simulink subsystem "PvtSubSys_VSM_ELK"  (R2020b)
settings: Solver=VariableStepAuto  StartTime=0.0  StopTime=10.0  RelTol=1e-3
values from neighbouring files (symbols this model uses):
  P_VSM_ELK_Curvature_R_Table : value not decoded    [ELK.sldd]
  P_VSM_ELK_Curvature_R_Table_Calibration : value not decoded    [ELK.sldd]
  P_VSM_ELK_Lane_Width_Table : value not decoded    [ELK.sldd]
  P_VSM_ELK_Lane_Width_Table_Calibration : value not decoded    [ELK.sldd]
  P_VSM_ELK_Lateral_Speed_Table : value not decoded    [ELK.sldd]
  P_VSM_ELK_Lateral_Speed_Table_Calibration : value not decoded    [ELK.sldd]
  P_VSM_ELK_OnComing_Lateral = 2.8    [ELK.sldd]
  P_VSM_ELK_OnComing_TTC = 3.0    [ELK.sldd]
  P_VSM_ELK_OverTaking_Lateral = 2.0    [ELK.sldd]
  P_VSM_ELK_OverTaking_TTC = 5.0    [ELK.sldd]
  P_VSM_ELK_Sensitive_Table : value not decoded    [ELK.sldd]
  P_VSM_ELK_Sensitive_Table_Calibration : value not decoded    [ELK.sldd]
  P_VSM_ELK_State_Absesp_enable = 1.0    [ELK.sldd]
  P_VSM_ELK_State_Accpedalrate_enable = 1.0    [ELK.sldd]
  P_VSM_ELK_State_Breakpressure_enable = 1.0    [ELK.sldd]
  P_VSM_ELK_State_DriverInputTrqValue_enable = 1.0    [ELK.sldd]
  P_VSM_ELK_State_Eps_enable = 1.0    [ELK.sldd]
  P_VSM_ELK_State_ESSSts_enable = 1.0    [ELK.sldd]
  P_VSM_ELK_State_Failsafe_enable = 1.0    [ELK.sldd]
  P_VSM_ELK_State_GEAR_enable = 1.0    [ELK.sldd]
  P_VSM_ELK_State_Handson_enable = 1.0    [ELK.sldd]
  P_VSM_ELK_State_Headingangle_enable = 1.0    [ELK.sldd]
  P_VSM_ELK_State_Lane_enable = 1.0    [ELK.sldd]
  P_VSM_ELK_State_LaneChange_enable = 1.0    [ELK.sldd]
  P_VSM_ELK_State_Lanecurve_enable = 1.0    [ELK.sldd]
  P_VSM_ELK_State_LateralAcce_enable = 1.0    [ELK.sldd]
  P_VSM_ELK_State_LongitudeAcc_enable = 1.0    [ELK.sldd]
  P_VSM_ELK_State_Overide_enable = 1.0    [ELK.sldd]
  P_VSM_ELK_State_Param_AngleOffset = 0.05    [ELK.sldd]
  P_VSM_ELK_State_Param_LaneTime : value not decoded    [ELK.sldd]
  P_VSM_ELK_State_Param_Oncoming = 0.55    [ELK.sldd]
  P_VSM_ELK_State_Param_OnTime : value not decoded    [ELK.sldd]
  P_VSM_ELK_State_Param_OutOffset = 0.15    [ELK.sldd]
  P_VSM_ELK_State_Param_Over = 0.55    [ELK.sldd]
  P_VSM_ELK_State_Param_OvTime : value not decoded    [ELK.sldd]
  P_VSM_ELK_State_Param_Speed : value not decoded    [ELK.sldd]
  P_VSM_ELK_State_SteerWheelAngle_enable = 1.0    [ELK.sldd]
  P_VSM_ELK_State_SteerWheelSpd_enable = 1.0    [ELK.sldd]
  P_VSM_ELK_State_TurnLight_enable = 1.0    [ELK.sldd]
  P_VSM_ELK_State_Vehspeed_enable = 1.0    [ELK.sldd]
  P_VSM_ELK_State_Yawsup_enable = 1.0    [ELK.sldd]
undefined symbols (not defined in the file or in its folder): ELKSTATE, P_Global_DxvRearBumper_m, P_Global_IEnvironment_RefPX_Front_Bumper, P_Global_IFV2Fwheel_Dx, P_Global_Vehicle_Length_m, P_Global_VehicleWidthMin_m, P_VSM_LSMC_SampleTime
libraries: simulink x167
(part 4 of 5)

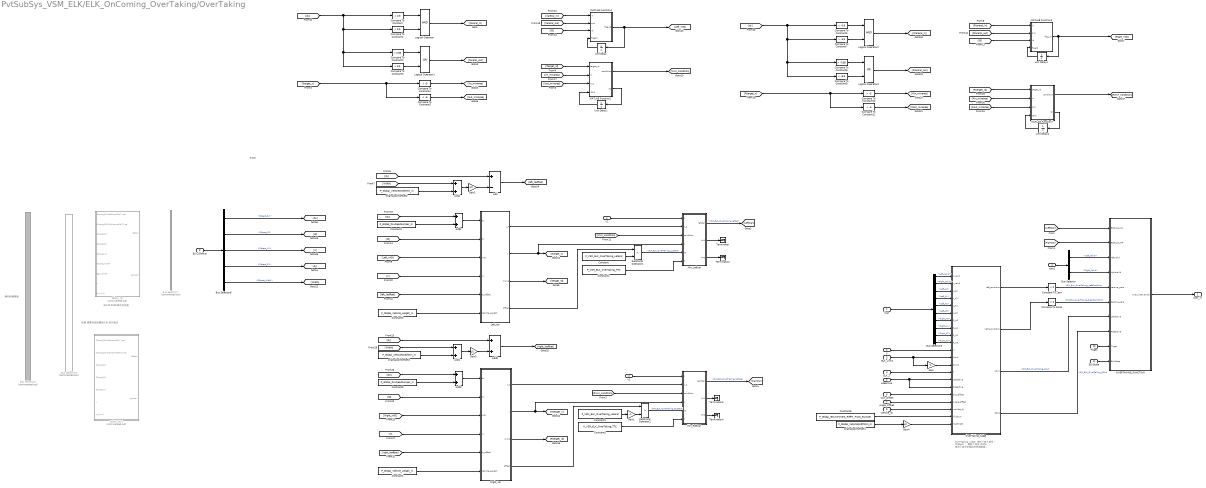
== system PvtSubSys_VSM_ELK/ELK_OnComing_OverTaking/OverTaking ==
  note: RSDS
  note: 横向距离限制
  note: 未对ttc和dtc做冗余处理
  note: 后期 需要对目标属性正负 进行验证
  note: OverTaking_Judge
      | 增加了输入信号：
      | ifv2bum；
      | 删除了信号
      | ifv2fw
      | 修改了自车车辆动态预测距离；
  ican : Inport
  V : Inport  Port=2
  ELK_Limit : Inport  Port=3
  ELK_T : Inport  Port=4
  Ldeactive : Inport  Port=5
  Out_Offset : Inport  Port=6
  Angle_Offset : Inport  Port=7
  ELK_ObjBus : Inport  Port=8
  Vehicle_dy : Inport  Port=9
  Triger : Inport  Port=10
  ELKState : Inport  Port=11
  Add : Sum  Inputs=+-
  Add{1..4,6} (5 alike) : Sum
  Bus Selector : BusSelector  OutputSignals=Left_Valid,Right_Valid
  Bus Selector3 : BusSelector  OutputSignals=Left_Valid,Right_Valid,Left_A0,Left_A1,Left_A2,Left_A3,Right_A0,Right_A1,Right_A2,Right_A3
  Bus Selector5 : BusSelector  Commented=on  OutputSignals=RSDSDx_RL,RSDSID_RL,RSDSV_RL,RSDSDy_RL,RSDSWth_RL,RSDSDx_RR,RSDSID_RR,RSDSV_RR,RSDSDy_RR,RSDSWth_RR
  Bus Selector6 : BusSelector  Commented=on  OutputSignals=ELK_Object_DX,ELK_Object_ID,ELK_Object_VX,ELK_Object_DY,ELK_Object_Width,ELK_Object_DX,ELK_Object_ID,ELK_Object_VX,ELK_Object_DY,ELK_Object_Width
  Bus Selector7 : BusSelector  Commented=on  OutputSignals=ELK_Object_DX,ELK_Object_ID,ELK_Object_VX,ELK_Object_DY,ELK_Object_Width
  Bus Selector8 : BusSelector  OutputSignals=Object_DX,Object_ID,Object_VX,Object_DY,Object_Width
  Compare To Constant : simulink/Logic and Bit Operations/Compare To Constant  relop=>  const=0.9  OutDataTypeStr=boolean
  Compare To Constant1 : simulink/Logic and Bit Operations/Compare To Constant  relop=<  const=5.5  OutDataTypeStr=boolean
  Compare To Constant10 : simulink/Logic and Bit Operations/Compare To Constant  relop=>  const=-5  OutDataTypeStr=boolean
  Compare To Constant11 : simulink/Logic and Bit Operations/Compare To Constant  relop=<  const=-6  OutDataTypeStr=boolean
  Compare To Constant2 : simulink/Logic and Bit Operations/Compare To Constant  relop=<  const=0.85  OutDataTypeStr=boolean
  Compare To Constant3 : simulink/Logic and Bit Operations/Compare To Constant  relop=>  const=6.5  OutDataTypeStr=boolean
  Compare To Constant4 : simulink/Logic and Bit Operations/Compare To Constant  relop=>  const=-5  OutDataTypeStr=boolean
  Compare To Constant5 : simulink/Logic and Bit Operations/Compare To Constant  relop=<  const=-6  OutDataTypeStr=boolean
  Compare To Constant6 : simulink/Logic and Bit Operations/Compare To Constant  relop=<  const=-0.9  OutDataTypeStr=boolean
  Compare To Constant7 : simulink/Logic and Bit Operations/Compare To Constant  relop=>  const=-5.5  OutDataTypeStr=boolean
  Compare To Constant8 : simulink/Logic and Bit Operations/Compare To Constant  relop=>  const=-0.85  OutDataTypeStr=boolean
  Compare To Constant9 : simulink/Logic and Bit Operations/Compare To Constant  relop=<  const=-6.5  OutDataTypeStr=boolean
  Compare To Zero : simulink/Logic and Bit Operations/Compare To Zero  relop=<  OutDataTypeStr=boolean
  Compare To Zero1 : simulink/Logic and Bit Operations/Compare To Zero  relop=>  OutDataTypeStr=boolean
  Constant : Constant  Value=P_VSM_ELK_OverTaking_Lateral
  Constant1 : Constant  Value=P_Global_Vehicle_Length_m
  Constant2 : Constant  Value=P_VSM_ELK_OverTaking_Lateral
  Constant3 : Constant  Value=P_Global_Vehicle_Length_m
  Constant4 : Constant  Value=P_VSM_ELK_OverTaking_TTC
  Constant5 : Constant  Value=P_VSM_ELK_OverTaking_TTC
  Constant6 : Constant  Value=P_Global_IEnvironment_RefPX_Front_Bumper
  Constant7 : Constant  Value=P_Global_DxvRearBumper_m
  Constant8 : Constant  Value=P_Global_DxvRearBumper_m
  Gain : Gain  Gain=-1
  Gain1 : Gain  Gain=-1
  Gain2 : Gain  Gain=1/2
  Gain3 : Gain  Gain=1/2
  Gain4 : Gain  Gain=1/2
  Left_tar : MATLAB Function  TreatAsAtomicUnit=on
  Logical Operator : Logic  AllPortsSameDT=off  OutDataTypeStr=boolean
  Logical Operator1 : Logic  Operator=OR  AllPortsSameDT=off  OutDataTypeStr=boolean
  Logical Operator2 : Logic  AllPortsSameDT=off  OutDataTypeStr=boolean
  Logical Operator3 : Logic  Operator=OR  AllPortsSameDT=off  OutDataTypeStr=boolean
  MATLAB Function1 : MATLAB Function  TreatAsAtomicUnit=on
  MATLAB Function3 : MATLAB Function  TreatAsAtomicUnit=on
  MATLAB Function4 : MATLAB Function  TreatAsAtomicUnit=on
  MATLAB Function7 : MATLAB Function  TreatAsAtomicUnit=on
  Min_Leftcar : MATLAB Function  TreatAsAtomicUnit=on
  Min_Reftcar : MATLAB Function  TreatAsAtomicUnit=on
  OVERTAKING_FUNCTION : Stateflow chart  TreatAsAtomicUnit=on
  OverTaking_Judge : MATLAB Function  TreatAsAtomicUnit=on
  Relational Operator1 : RelationalOperator  Operator=<  OutDataTypeStr=boolean  RndMeth=Simplest
  Relational Operator2 : RelationalOperator  Operator=>  OutDataTypeStr=boolean  RndMeth=Simplest
  Right_tar : MATLAB Function  TreatAsAtomicUnit=on
  Select_tar : MATLAB Function  Commented=on  TreatAsAtomicUnit=on
  Select_tar2 : MATLAB Function  Commented=on  TreatAsAtomicUnit=on
  Terminator{,2..4} (4 alike) : Terminator
  Unit Delay{,1..2,4} (4 alike) : UnitDelay  InitialCondition=uint8(0)  SampleTime=-1  HasFrameUpgradeWarning=on
  V1 : InportShadow  Port=2
  V2 : InportShadow  Port=2
  ican1 : InportShadow
  originalpointoffset1 : Constant  Value=P_Global_VehicleWidthMin_m
  originalpointoffset2 : Constant  Value=P_Global_VehicleWidthMin_m
  originalpointoffset3 : Constant  Value=P_Global_VehicleWidthMin_m
  "over_in " : Outport
  wires:
  Bus Selector/2 -> OVERTAKING_FUNCTION/4(rightvalid)  "<Right_Valid>"
  Bus Selector/1 -> OVERTAKING_FUNCTION/3(leftvalid)  "<Left_Valid>"
  ican1/1 -> Bus Selector/1
  Bus Selector3/10 -> OverTaking_Judge/10(R_A3)  "<Right_A3>"
  Bus Selector3/9 -> OverTaking_Judge/9(R_A2)  "<Right_A2>"
  Bus Selector3/8 -> OverTaking_Judge/8(R_A1)  "<Right_A1>"
  Bus Selector3/7 -> OverTaking_Judge/7(R_A0)  "<Right_A0>"
  Bus Selector3/6 -> OverTaking_Judge/6(L_A3)  "<Left_A3>"
  Bus Selector3/5 -> OverTaking_Judge/5(L_A2)  "<Left_A2>"
  Bus Selector3/4 -> OverTaking_Judge/4(L_A1)  "<Left_A1>"
  Bus Selector3/3 -> OverTaking_Judge/3(L_A0)  "<Left_A0>"
  Bus Selector3/2 -> OverTaking_Judge/2(r_valid)  "<Right_Valid>"
  Bus Selector3/1 -> OverTaking_Judge/1(l_valid)  "<Left_Valid>"
  Gain3/1 -> Add6/2
  [Width] -> Add1/1
  [V] -> Right_tar/4(vx)
  [Dx] -> Add3/1
  [dy] -> Add6/1
  [ID] -> Right_tar/2(id)
  [V] -> Left_tar/4(vx)
  Bus Selector8/3 -> [V]  "<Object_VX>"
  [Dx] -> Add2/1
  Bus Selector8/1 -> [Dx]  "<Object_DX>"
  [ID] -> Left_tar/2(id)
  Bus Selector8/2 -> [ID]  "<Object_ID>"
  [Width] -> Add4/1
  Bus Selector8/5 -> [Width]  "<Object_Width>"
  Bus Selector8/4 -> [dy]  "<Object_DY>"
  Unit Delay2/1 -> MATLAB Function7/4(IDk1)
  MATLAB Function7/2(ID) -> Unit Delay2/1
  Unit Delay1/1 -> MATLAB Function1/4(IDk1)
  MATLAB Function1/2(ID) -> Unit Delay1/1
  Unit Delay/1 -> MATLAB Function4/4(flagk1)
  MATLAB Function4/1(flag_id) -> Unit Delay/1, [Left_inID]
  Unit Delay4/1 -> MATLAB Function3/4(flagk1)
  Gain1/1 -> Relational Operator2/2
  Constant2/1 -> Gain1/1
  Constant/1 -> Relational Operator1/2
  Angle_Offset/1 -> OverTaking_Judge/18(Angle_Offset)
  Out_Offset/1 -> OverTaking_Judge/17(Out_Offset)
  OverTaking_Judge/4(ROut) -> OVERTAKING_FUNCTION/8(Rdeactive)  "VSM_ELK_OverTaking_ROut"
  OverTaking_Judge/3(LOut) -> OVERTAKING_FUNCTION/7(Ldeactive)  "VSM_ELK_OverTaking_LOut"
  OverTaking_Judge/2(right_condition) -> Compare To Zero1/1
  OverTaking_Judge/1(left_condition) -> Compare To Zero/1
  [right_laoffset] -> Right_tar/5(la_offset)
  [left_laoffset] -> Left_tar/5(la_offset)
  Relational Operator2/1 -> Min_Reftcar/5(la)  "VSM_ELK_OverTaking_RLateral"
  Right_tar/4(offset) -> Relational Operator2/1
  Relational Operator1/1 -> Min_Leftcar/5(la)  "VSM_ELK_OverTaking_LLateral"
  Left_tar/4(offset) -> Relational Operator1/1
  Add6/1 -> [right_laoffset]
  Add1/1 -> Gain3/1
  Add/1 -> [left_laoffset]
  Constant8/1 -> Add3/2
  Add3/1 -> Right_tar/1(dx)
  Constant3/1 -> Left_tar/6(Vehicle_Length)
  Add2/1 -> Left_tar/1(dx)
  [ID] -> MATLAB Function3/3(id)
  Compare To Constant6/1 -> Logical Operator2/1
  [Rin_minarea] -> MATLAB Function7/2(in)
  MATLAB Function3/1(flag_id) -> Unit Delay4/1, [Right_inID]
  [Rterget_id] -> MATLAB Function7/1(target_id)
  [Rout_minarea] -> MATLAB Function7/3(out)
  MATLAB Function7/1(condition) -> [Rmin_condition]
  Compare To Constant7/1 -> Logical Operator2/2
  Compare To Constant9/1 -> Logical Operator3/2
  Logical Operator2/1 -> [Rlareral_in]
  Compare To Constant11/1 -> [Rout_minarea]
  Compare To Constant8/1 -> Logical Operator3/1
  [Rterget_x] -> Compare To Constant11/1, Compare To Constant10/1
  [dy] -> Compare To Constant9/1, Compare To Constant8/1, Compare To Constant7/1, Compare To Constant6/1
  Logical Operator3/1 -> [Rlareral_out]
  Compare To Constant10/1 -> [Rin_minarea]
  [Rlareral_in] -> MATLAB Function3/1(in)
  [Rlareral_out] -> MATLAB Function3/2(out)
  [Rmin_condition] -> Min_Reftcar/3(condition)
  Right_tar/2(x) -> Min_Reftcar/4(x), [Rterget_x]
  Right_tar/3(minid) -> [Rterget_id]
  V2/1 -> Min_Reftcar/1(v)
  [Right_inID] -> Right_tar/3(inID)
  Right_tar/1(v_t) -> Min_Reftcar/2(v_t)
  Min_Reftcar/1(rightcar) -> [RightCar]  "VSM_ELK_OverTaking_rightcar"
  Min_Reftcar/2(Vo1) -> Terminator3/1
  Min_Reftcar/3(TTC) -> Terminator4/1
  Min_Leftcar/3(TTC) -> Terminator2/1
  Min_Leftcar/2(Vo1) -> Terminator/1
  Min_Leftcar/1(leftcar) -> [LeftCar]  "VSM_ELK_OverTaking_leftcar"
  [llareral_out] -> MATLAB Function4/2(out)
  Left_tar/1(v_t) -> Min_Leftcar/2(v_t)
  [llareral_in] -> MATLAB Function4/1(in)
  [Left_inID] -> Left_tar/3(inID)
  V1/1 -> Min_Leftcar/1(v)
  Compare To Constant4/1 -> [lin_minarea]
  Logical Operator1/1 -> [llareral_out]
  [dy] -> Compare To Constant/1, Compare To Constant3/1, Compare To Constant2/1, Compare To Constant1/1
  [lterget_x] -> Compare To Constant4/1, Compare To Constant5/1
  Compare To Constant2/1 -> Logical Operator1/1
  Compare To Constant5/1 -> [lout_minarea]
  Logical Operator/1 -> [llareral_in]
  Compare To Constant3/1 -> Logical Operator1/2
  Left_tar/3(minid) -> [lterget_id]
  Compare To Constant1/1 -> Logical Operator/2
  [dy] -> Add/1
  MATLAB Function1/1(condition) -> [lmin_condition]
  Left_tar/2(x) -> Min_Leftcar/4(x), [lterget_x]
  [lout_minarea] -> MATLAB Function1/3(out)
  [lterget_id] -> MATLAB Function1/1(target_id)
  [lin_minarea] -> MATLAB Function1/2(in)
  Compare To Constant/1 -> Logical Operator/1
  [ID] -> MATLAB Function4/3(id)
  [lmin_condition] -> Min_Leftcar/3(condition)
  [LeftCar] -> OVERTAKING_FUNCTION/1(BSDLCA_WL)
  [RightCar] -> OVERTAKING_FUNCTION/2(BSDLCA_WR)
  OVERTAKING_FUNCTION/1(over_intervention) -> "over_in "/1
  ican/1 -> Bus Selector3/1
  ELK_T/1 -> OverTaking_Judge/14(T)
  ELK_Limit/1 -> Gain/1, OverTaking_Judge/12(Limit)
  V/1 -> OverTaking_Judge/11(V)
  Gain/1 -> OverTaking_Judge/13(Rlimit)
  Add4/1 -> Gain2/1
  Gain2/1 -> Add/2
  Vehicle_dy/1 -> OverTaking_Judge/19(vehicle_dy)
  Compare To Zero/1 -> OVERTAKING_FUNCTION/5(Lactive_para)  "VSM_ELK_OverTaking_LeftCondition"
  Compare To Zero1/1 -> OVERTAKING_FUNCTION/6(Ractive_para)  "VSM_ELK_OverTaking_RightCondition"
  Constant4/1 -> Min_Leftcar/6(T)
  Constant5/1 -> Min_Reftcar/6(T)
  originalpointoffset1/1 -> Gain4/1
  ELK_ObjBus/1 -> Bus Selector8/1
  Gain4/1 -> OverTaking_Judge/21(HalfWidth)
  Constant6/1 -> OverTaking_Judge/20(ifv2bum)
  originalpointoffset2/1 -> Add4/2
  originalpointoffset3/1 -> Add1/2
  Ldeactive/1 -> OverTaking_Judge/16(Rdeactive), OverTaking_Judge/15(Ldeactive)
  Triger/1 -> OVERTAKING_FUNCTION/9(Triger)
  ELKState/1 -> OVERTAKING_FUNCTION/10(ELKState)
  Constant7/1 -> Add2/2
  Constant1/1 -> Right_tar/6(Vehicle_Length)

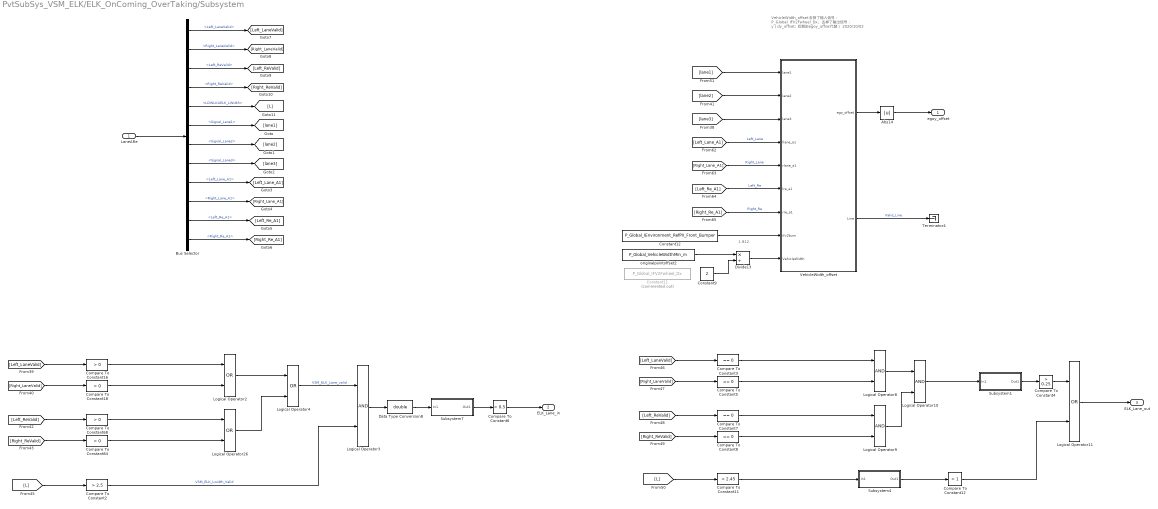
== system PvtSubSys_VSM_ELK/ELK_OnComing_OverTaking/Subsystem ==
  note: 1.812
  note: VehicleWidth_offset
      | 去掉了输入信号：
      | P_Global_IFV2Fwheel_Dx；
      | 去掉了输出信号：
      | y（dy_offset；后期由egoy_offset代替）
      | 2020/10/02
  LaneARe : Inport
  Abs14 : Abs
  Bus Selector : BusSelector  OutputSignals=Left_LaneValid,Right_LaneValid,Left_ReValid,Right_ReValid,LDWLKAELK_LWidth,Signal_Lane1,Signal_Lane2,Signal_Lane3,Left_Lane_A1,Right_Lane_A1,Left_Re_A1,Right_Re_A1
  Compare To Constant11 : simulink/Logic and Bit Operations/Compare To Constant  relop=<  const=2.45  OutDataTypeStr=boolean
  Compare To Constant12 : simulink/Logic and Bit Operations/Compare To Constant  relop=>  const=1  OutDataTypeStr=boolean
  Compare To Constant{16,18,68,84} (4 alike) : simulink/Logic and Bit Operations/Compare To Constant  relop=>  const=0  OutDataTypeStr=boolean
  Compare To Constant2 : simulink/Logic and Bit Operations/Compare To Constant  relop=>  const=2.5  OutDataTypeStr=boolean
  Compare To Constant{3,5,7..8} (4 alike) : simulink/Logic and Bit Operations/Compare To Constant  relop===  const=0  OutDataTypeStr=boolean
  Compare To Constant4 : simulink/Logic and Bit Operations/Compare To Constant  relop=>  const=0.25  OutDataTypeStr=boolean
  Compare To Constant6 : simulink/Logic and Bit Operations/Compare To Constant  relop=>  const=0.5  OutDataTypeStr=boolean
  Constant11 : Constant  Commented=on  Value=P_Global_IFV2Fwheel_Dx
  Constant12 : Constant  Value=P_Global_IEnvironment_RefPX_Front_Bumper
  Constant9 : Constant  Value=2  OutDataTypeStr=single
  Data Type Conversion8 : DataTypeConversion  OutDataTypeStr=double
  Divide13 : Product  Inputs=*/
  Logical Operator{3,8..10} (4 alike) : Logic  AllPortsSameDT=off  OutDataTypeStr=boolean
  Logical Operator{2,4,11,26} (4 alike) : Logic  Operator=OR  AllPortsSameDT=off  OutDataTypeStr=boolean
  Subsystem1 : Subsystem  mask{Ts=P_VSM_LSMC_SampleTime, Max=10}
      mask prompts: Ts "Sample Time:"; Max "Max Limit:"
      mask Display:
      | Ts=get_param(gcb,'Ts');
      | Max=get_param(gcb,'Max');
      | disp(['Ts:' Ts '\n' 'Max:' Max ]);
  Subsystem4 : Subsystem  mask{Ts=P_VSM_LSMC_SampleTime, Max=10}
      mask prompts: Ts "Sample Time:"; Max "Max Limit:"
      mask Display:
      | Ts=get_param(gcb,'Ts');
      | Max=get_param(gcb,'Max');
      | disp(['Ts:' Ts '\n' 'Max:' Max ]);
  Subsystem7 : Subsystem  mask{Ts=P_VSM_LSMC_SampleTime, Max=10}
      mask prompts: Ts "Sample Time:"; Max "Max Limit:"
      mask Display:
      | Ts=get_param(gcb,'Ts');
      | Max=get_param(gcb,'Max');
      | disp(['Ts:' Ts '\n' 'Max:' Max ]);
  Terminator4 : Terminator
  VehicleWidth_offset : MATLAB Function  TreatAsAtomicUnit=on
  originalpointoffset2 : Constant  Value=P_Global_VehicleWidthMin_m
  egoy_offset : Outport
  ELK_Lane_in : Outport  Port=2
  ELK_Lane_out : Outport  Port=3
  wires:
  Bus Selector/12 -> [Right_Re_A1]  "<Right_Re_A1>"
  Bus Selector/11 -> [Left_Re_A1]  "<Left_Re_A1>"
  Bus Selector/10 -> [Right_Lane_A1]  "<Right_Lane_A1>"
  Bus Selector/9 -> [Left_Lane_A1]  "<Left_Lane_A1>"
  Bus Selector/8 -> [lane3]  "<Signal_Lane3>"
  Bus Selector/6 -> [lane1]  "<Signal_Lane1>"
  Bus Selector/7 -> [lane2]  "<Signal_Lane2>"
  Bus Selector/5 -> [L]  "<LDWLKAELK_LWidth>"
  Bus Selector/1 -> [Left_LaneValid]  "<Left_LaneValid>"
  Bus Selector/2 -> [Right_LaneValid]  "<Right_LaneValid>"
  Bus Selector/4 -> [Right_ReValid]  "<Right_ReValid>"
  Bus Selector/3 -> [Left_ReValid]  "<Left_ReValid>"
  Logical Operator26/1 -> Logical Operator4/2
  Logical Operator4/1 -> Logical Operator3/1  "VSM_ELK_Lane_valid"
  Compare To Constant18/1 -> Logical Operator2/2
  Data Type Conversion8/1 -> Subsystem7/1(In1)
  [Right_ReValid] -> Compare To Constant8/1
  [Right_LaneValid] -> Compare To Constant5/1
  [Right_LaneValid] -> Compare To Constant18/1
  [Left_LaneValid] -> Compare To Constant16/1
  [Right_ReValid] -> Compare To Constant84/1
  Subsystem1/1(Out1) -> Compare To Constant4/1
  originalpointoffset2/1 -> Divide13/1
  [L] -> Compare To Constant11/1
  [Left_LaneValid] -> Compare To Constant3/1
  Compare To Constant68/1 -> Logical Operator26/1
  Compare To Constant16/1 -> Logical Operator2/1
  Compare To Constant5/1 -> Logical Operator8/2
  Compare To Constant12/1 -> Logical Operator11/2
  VehicleWidth_offset/2(Line) -> Terminator4/1  "Valid_Line"
  Compare To Constant2/1 -> Logical Operator3/2  "VSM_ELK_Lwidth_Valid"
  Constant9/1 -> Divide13/2
  [Right_Re_A1] -> VehicleWidth_offset/7(rre_a1)  "Right_Re"
  Constant12/1 -> VehicleWidth_offset/8(ifv2bum)
  Logical Operator9/1 -> Logical Operator10/2
  Logical Operator11/1 -> ELK_Lane_out/1
  Compare To Constant3/1 -> Logical Operator8/1
  Subsystem7/1(Out1) -> Compare To Constant6/1
  [Left_ReValid] -> Compare To Constant68/1
  [Left_ReValid] -> Compare To Constant7/1
  Compare To Constant6/1 -> ELK_Lane_in/1
  VehicleWidth_offset/1(ego_offset) -> Abs14/1
  Subsystem4/1(Out1) -> Compare To Constant12/1
  Logical Operator10/1 -> Subsystem1/1(In1)
  [lane2] -> VehicleWidth_offset/2(lane2)
  [lane3] -> VehicleWidth_offset/3(lane3)
  Compare To Constant11/1 -> Subsystem4/1(In1)
  Logical Operator3/1 -> Data Type Conversion8/1
  Logical Operator2/1 -> Logical Operator4/1
  Compare To Constant7/1 -> Logical Operator9/1
  Compare To Constant8/1 -> Logical Operator9/2
  [Left_Lane_A1] -> VehicleWidth_offset/4(llane_a1)  "Left_Lane"
  [lane1] -> VehicleWidth_offset/1(lane1)
  [L] -> Compare To Constant2/1
  Abs14/1 -> egoy_offset/1
  Divide13/1 -> VehicleWidth_offset/9(VehicleWidth)
  [Left_Re_A1] -> VehicleWidth_offset/6(lre_a1)  "Left_Re"
  Compare To Constant84/1 -> Logical Operator26/2
  Compare To Constant4/1 -> Logical Operator11/1
  [Right_Lane_A1] -> VehicleWidth_offset/5(rlane_a1)  "Right_Lane"
  Logical Operator8/1 -> Logical Operator10/1
  LaneARe/1 -> Bus Selector/1

== system PvtSubSys_VSM_ELK/ELK_OnComing_OverTaking/Subsystem2 ==
  In1 : Inport
  Add : Sum
  Constant : Constant  Value=Ts
  Constant1 : Constant  Value=0
  Constant2 : Constant  Value=Max
  Max : MinMax  Inputs=2
  Switch : Switch  Criteria=u2 ~= 0
  Unit Delay : UnitDelay  SampleTime=-1  HasFrameUpgradeWarning=on
  Out1 : Outport
  wires:
  Unit Delay/1 -> Add/1
  In1/1 -> Switch/2
  Constant/1 -> Add/2
  Constant1/1 -> Switch/3
  Add/1 -> Switch/1
  Max/1 -> Unit Delay/1, Out1/1
  Constant2/1 -> Max/2
  Switch/1 -> Max/1

== system PvtSubSys_VSM_ELK/ELK_OnComing_OverTaking/Subsystem3 ==
  In1 : Inport
  Add : Sum
  Constant : Constant  Value=Ts
  Constant1 : Constant  Value=0
  Constant2 : Constant  Value=Max
  Max : MinMax  Inputs=2
  Switch : Switch  Criteria=u2 ~= 0
  Unit Delay : UnitDelay  SampleTime=-1  HasFrameUpgradeWarning=on
  Out1 : Outport
  wires:
  Switch/1 -> Max/1
  Constant2/1 -> Max/2
  Max/1 -> Out1/1, Unit Delay/1
  Add/1 -> Switch/1
  Constant1/1 -> Switch/3
  Constant/1 -> Add/2
  In1/1 -> Switch/2
  Unit Delay/1 -> Add/1

== system PvtSubSys_VSM_ELK/ELK_OnComing_OverTaking/Subsystem/Subsystem1 ==
  In1 : Inport
  Add : Sum
  Constant : Constant  Value=Ts
  Constant1 : Constant  Value=0
  Constant2 : Constant  Value=Max
  Max : MinMax  Inputs=2
  Switch : Switch  Criteria=u2 ~= 0
  Unit Delay : UnitDelay  SampleTime=-1  HasFrameUpgradeWarning=on
  Out1 : Outport
  wires:
  Switch/1 -> Max/1
  Constant2/1 -> Max/2
  Max/1 -> Out1/1, Unit Delay/1
  Add/1 -> Switch/1
  Constant1/1 -> Switch/3
  Constant/1 -> Add/2
  In1/1 -> Switch/2
  Unit Delay/1 -> Add/1

== system PvtSubSys_VSM_ELK/ELK_OnComing_OverTaking/Subsystem/Subsystem4 ==
  In1 : Inport
  Add : Sum
  Constant : Constant  Value=Ts
  Constant1 : Constant  Value=0
  Constant2 : Constant  Value=Max
  Max : MinMax  Inputs=2
  Switch : Switch  Criteria=u2 ~= 0
  Unit Delay : UnitDelay  SampleTime=-1  HasFrameUpgradeWarning=on
  Out1 : Outport
  wires:
  Unit Delay/1 -> Add/1
  In1/1 -> Switch/2
  Constant/1 -> Add/2
  Constant1/1 -> Switch/3
  Add/1 -> Switch/1
  Max/1 -> Unit Delay/1, Out1/1
  Constant2/1 -> Max/2
  Switch/1 -> Max/1

== system PvtSubSys_VSM_ELK/ELK_OnComing_OverTaking/Subsystem/Subsystem7 ==
  In1 : Inport
  Add : Sum
  Constant : Constant  Value=Ts
  Constant1 : Constant  Value=0
  Constant2 : Constant  Value=Max
  Max : MinMax  Inputs=2
  Switch : Switch  Criteria=u2 ~= 0
  Unit Delay : UnitDelay  SampleTime=-1  HasFrameUpgradeWarning=on
  Out1 : Outport
  wires:
  Switch/1 -> Max/1
  Constant2/1 -> Max/2
  Max/1 -> Out1/1, Unit Delay/1
  Add/1 -> Switch/1
  Constant1/1 -> Switch/3
  Constant/1 -> Add/2
  In1/1 -> Switch/2
  Unit Delay/1 -> Add/1

== matlab function PvtSubSys_VSM_ELK/ELK_Condition/State_TurnLight2 ==
  data: leftlight input; rightlight input; lane input; state output; out output; leftk1 input; left output; rightk1 input; right output
function [state,out,left,right] = fcn(leftlight,rightlight,lane,leftk1,rightk1)
left=0;
right=0;
if leftlight==1 && lane==1  % left alone
    state=1;
    out=0;
    left=1;
elseif lane==1 && leftk1==1  
    state=0;
    out=0;
    left=1;
elseif lane ==1
    state=0;
    out=1;
    left=0;
elseif rightlight==1 && lane==2
    state=1;
    out=0;
    right=1;
elseif lane==2 && rightk1==1
    state=0;
    out=0;
    right=1;
elseif lane ==2
    state=0;
    out=1;
    right=0;
    
else
    state=0;
    out=0;
    left=0;
end

== matlab function PvtSubSys_VSM_ELK/ELK_OnComing_OverTaking/OnComing/MATLAB Function1 ==
  data: in input; flag_id output uint8; out input; id input; flagk1 input
function flag_id = fcn(in,out,id,flagk1)
flag_id=uint8(zeros(8,1));
for i=1:8
   if in(i)>0
        flag_id(i)=id(i);
   elseif in(i)==0 && out(i)==0
       for j=1:8
       if flagk1(j)==id(i)
           flag_id(i)=id(i);
       end
       end
   elseif out(i)>0
       flag_id(i)=uint8(0);
   end
end

== matlab function PvtSubSys_VSM_ELK/ELK_OnComing_OverTaking/OnComing/MATLAB Function3 ==
  data: in input; flag_id output uint8; out input; id input; flagk1 input
function flag_id = fcn(in,out,id,flagk1)
flag_id=uint8(zeros(8,1));
for i=1:8
   if in(i)>0
        flag_id(i)=id(i);
   elseif in(i)==0 && out(i)==0
       for j=1:8
       if flagk1(j)==id(i)
           flag_id(i)=id(i);
       end
       end
   elseif out(i)>0
       flag_id(i)=uint8(0);
   end
end

== matlab function PvtSubSys_VSM_ELK/ELK_OnComing_OverTaking/OverTaking/MATLAB Function3 ==
  data: in input; flag_id output uint8; out input; id input; flagk1 input
function flag_id = fcn(in,out,id,flagk1)
flag_id=uint8(zeros(8,1));
for i=1:8
   if in(i)>0
        flag_id(i)=id(i);
   elseif in(i)==0 && out(i)==0
       for j=1:8
       if flagk1(j)==id(i)
           flag_id(i)=id(i);
       end
       end
   elseif out(i)>0
       flag_id(i)=uint8(0);
   end
end

== matlab function PvtSubSys_VSM_ELK/ELK_OnComing_OverTaking/OverTaking/MATLAB Function4 ==
  data: in input; flag_id output uint8; out input; id input; flagk1 input
function flag_id = fcn(in,out,id,flagk1)
flag_id=uint8(zeros(8,1));
for i=1:8
   if in(i)>0
        flag_id(i)=id(i);
   elseif in(i)==0 && out(i)==0
       for j=1:8
       if flagk1(j)==id(i)
           flag_id(i)=id(i);
       end
       end
   elseif out(i)>0
       flag_id(i)=uint8(0);
   end
end

== matlab function PvtSubSys_VSM_ELK/ELK_OnComing_OverTaking/Subsystem/VehicleWidth_offset ==
  data: lane1 input; ego_offset output single; lane2 input; lane3 input; llane_a1 input; rlane_a1 input; lre_a1 input; rre_a1 input; Line output single; ifv2bum input; VehicleWidth input
function [ego_offset,Line] = fcn(lane1,lane2,lane3,llane_a1,rlane_a1,lre_a1,rre_a1,ifv2bum,VehicleWidth)
if lane1==single(1)||lane2==single(1)||lane3==single(1) % left
    a1=atan(llane_a1);
%     y=(0.9+ifv2fw*tan(a1))*cos(a1);
    Line=single(1);    
    if a1>0
        ego_offset=single((VehicleWidth+ifv2bum*tan(a1))*cos(a1));
    else
        ego_offset=VehicleWidth;
    end
elseif lane1==single(2)||lane2==single(2)||lane3==single(2) % right
    a2=atan(rlane_a1);
%     y=(0.9-ifv2fw*tan(a2))*cos(a2);
    Line=single(2);
    if a2<0
        ego_offset=single((VehicleWidth-ifv2bum*tan(a2))*cos(a2));
    else
        ego_offset=VehicleWidth;
    end
elseif lane1==single(3)||lane2==single(3)||lane3==single(3)
    a3=atan(lre_a1);
%     y=(0.9+ifv2fw*tan(a3))*cos(a3);
    Line=single(3);
    if a3>0
      ego_offset=single((VehicleWidth+ifv2bum*tan(a3))*cos(a3));
    else
      ego_offset=VehicleWidth;
    end
elseif lane1==single(4)||lane2==single(4)||lane3==single(4)
    a4=atan(rre_a1);
%     y=(0.9-ifv2fw*tan(a4))*cos(a4);
    Line=single(4);
    if a4<0
        ego_offset=single((VehicleWidth-ifv2bum*tan(a4))*cos(a4));
    else
        ego_offset=VehicleWidth;
    end

else
%     y=0.9;
    Line=single(0);
    ego_offset=VehicleWidth;
    
        
end

== matlab function PvtSubSys_VSM_ELK/ELK_Condition/MATLAB Function ==
  data: LeftChangefg input; y output; RightChangefg input; Ldy input; Rdy input; Lfgk1 input; Lfg output; Rfgk1 input; Rfg output
function [y,Lfg,Rfg] = fcn(LeftChangefg,RightChangefg,Ldy,Rdy,Lfgk1,Rfgk1)
y=1;
Lfg=0;
Rfg=0;
if LeftChangefg>0
    Lfg=1;
    y=0;
elseif Lfgk1>0
    Lfg=1;
    y=0;
    if Rdy>0
        Lfg=0;
        y=1;
    end
    
end

if RightChangefg>0
    Rfg=1;
    y=0;
elseif Rfgk1>0
    Rfg=1;
    y=0;
    if Ldy>0
        Rfg=0;
        y=1;
    end
    
end

== stateflow chart PvtSubSys_VSM_ELK/ELK_State ==
  state MAINST_ON
    state SUBST_IDLE
      en:state=ELKSTATE.ELK_IDLE;
    state SUBST_ACTIVE
      state SUBSTLEFT_ACTIVE
        en:state=Left;
        SUBSTLEFT_ACTIVE -> (junction 125) [order 1]
        (junction 125) -> SUBSTLEFT_ACTIVE [order 2] : {warn=0;L=0;}
        (junction 125) -> SUBSTLEFT_ACTIVE [order 1] : [Leftwarn]{warn=1;L=L+1;}
      state SUBSTRIGHT_ACTIVE
        en:state=Right;
        SUBSTRIGHT_ACTIVE -> (junction 131) [order 1]
        (junction 131) -> SUBSTRIGHT_ACTIVE [order 2] : {warn=0;R=0;}
        (junction 131) -> SUBSTRIGHT_ACTIVE [order 1] : [Rightwarn]{warn=1;R=R+1;}
      (junction 61) -> SUBSTLEFT_ACTIVE [order 1] : [IN_L==true]
      (junction 61) -> SUBSTRIGHT_ACTIVE [order 2] : [IN_R==true]
    state SUBST_READY
      en:state=ELKSTATE.ELK_READY;
      warn=0;
      L=0;
      R=0;
    (default) -> SUBST_IDLE
    SUBST_IDLE -> SUBST_READY : [InCondition]
    SUBST_READY -> SUBST_IDLE [order 1] : [OutCondition]
    SUBST_ACTIVE -> SUBST_IDLE : [OutCondition]{warn=0;L=0;R=0;}
    SUBSTLEFT_ACTIVE -> SUBST_READY [order 1] : [Out_Common||IN_L==false||L>3*50]
    SUBST_READY -> (junction 61) [order 2] : [Common]
    SUBSTRIGHT_ACTIVE -> SUBST_READY [order 1] : [Out_Common||IN_R==false||R>3*50]
  state MAINST_OFF
    en:state=ELKSTATE.ELK_OFF;
  state MAINST_ERROR
    en:state=ELKSTATE.ELK_ERROR;
  (default) -> MAINST_OFF
  MAINST_OFF -> MAINST_ON [order 1] : [ELKSwitch==true && VehConfigELK==1]
  MAINST_ON -> MAINST_OFF [order 2] : [ELKSwitch==false]
  MAINST_OFF -> MAINST_ERROR [order 2] : [ELKSwitch==true&&ErrorDetected==1 && VehConfigELK==1]
  MAINST_ERROR -> MAINST_OFF [order 1] : [ELKSwitch==false]
  MAINST_ON -> MAINST_ERROR [order 1] : [ErrorDetected==1]
  MAINST_ERROR -> MAINST_ON [order 2] : [ELKSwitch==true&&ErrorDetected==0]
  data: ELKSwitch input boolean; VehConfigELK input uint8; ErrorDetected input; InCondition input boolean; OutCondition input boolean; Common input; Out_Common input; Left input; Right input; IN_L input boolean; IN_R input boolean; state output Enum: ELKSTATE =ELKSTATE.ELK_OFF; Ac_time local =0; warn output single; L local =0; R local =0; Leftwarn input; Rightwarn input

== matlab function PvtSubSys_VSM_ELK/ELK_OnComing_OverTaking/CalcEgoVehMove ==
  data: ON_dDeltaX output single size=1; On_T input single size=1; Over_T input; Vego input single size=1; Kap input single size=1; alpSideSlipAngle input single size=1; ON_dDeltaY output single size=1; OVER_dDeltaX output single size=1; OVER_dDeltaY output single size=1
function [ON_dDeltaX,ON_dDeltaY,OVER_dDeltaX,OVER_dDeltaY] = EgoVehicleMovement(On_T,Over_T,Vego,Kap,alpSideSlipAngle)
%#codegen
if abs(Kap)<0.00001
    ON_dDeltaX = Vego*On_T;
    ON_dDeltaY = single(0);
else
    t_Psi = asin(Kap*Vego*On_T);
    SinOfPsi = sin(t_Psi);
    t_dDeltaXTemp = SinOfPsi/Kap;
    t_dDeltaYTemp = single(2*(sin(t_Psi/2)*sin(t_Psi/2))/Kap);
    ON_dDeltaX = cos(alpSideSlipAngle)*t_dDeltaXTemp - sin(alpSideSlipAngle)*t_dDeltaYTemp;
    ON_dDeltaY = sin(alpSideSlipAngle)*t_dDeltaXTemp + cos(alpSideSlipAngle)*t_dDeltaYTemp;
end

if abs(Kap)<0.00001
    OVER_dDeltaX = Vego*Over_T;
    OVER_dDeltaY = single(0);

else
    t_Psi = asin(Kap*Vego*Over_T);
    SinOfPsi = sin(t_Psi);
    t_dDeltaXTemp = SinOfPsi/Kap;
    t_dDeltaYTemp = single(2*(sin(t_Psi/2)*sin(t_Psi/2))/Kap);
    OVER_dDeltaX = cos(alpSideSlipAngle)*t_dDeltaXTemp - sin(alpSideSlipAngle)*t_dDeltaYTemp;
    OVER_dDeltaY = sin(alpSideSlipAngle)*t_dDeltaXTemp + cos(alpSideSlipAngle)*t_dDeltaYTemp;
end

== matlab function PvtSubSys_VSM_ELK/ELK_OnComing_OverTaking/MATLAB Function ==
  data: LKAState input uint8; RE_Intervene output single; Lre input; Rre input
function RE_Intervene = fcn(LKAState,Lre,Rre)

if LKAState==uint8(4) && Lre==true
    RE_Intervene=single(1); % left
elseif LKAState==uint8(5) && Rre==true
    RE_Intervene=single(2);
else
    RE_Intervene=single(0);
end

== matlab function PvtSubSys_VSM_ELK/ELK_OnComing_OverTaking/MATLAB Function2 ==
  data: Left output Enum: ELKSTATE; Re input; Right output Enum: ELKSTATE; OnComing input; OverTaking input; IN_L output; IN_R output; Line_type output; Switch output; flag_On output; flag_Over output; flag_re output; flag_Onk1 input single; flag_Overk1 input single; flag_rek1 input single
function [Left,Right,IN_L,IN_R,Line_type,Switch,flag_On,flag_Over,flag_re] =f2(Re,OnComing,OverTaking,flag_Onk1,flag_Overk1,flag_rek1)
%Switch = 1 road edge on;  2: oncoming on;  3 = overtaking on 
   Left=ELKSTATE.ELK_OFF;
    Right=ELKSTATE.ELK_OFF;  
    IN_L=false;
    IN_R=false;
    Switch=single(0);
    Line_type=single(0);
    flag_On=single(0);
    flag_Over=single(0);
    flag_re=single(0);

if OnComing > 0 && flag_Overk1==single(0) && flag_rek1==single(0)
       Switch=single(2);
       Line_type=single(1);   % line
       flag_On=single(1);
    if OnComing==single(1)
        Left=ELKSTATE.ELK_ONCOMING_LEFT;
        IN_L=true;
    elseif OnComing==single(2)
        Right=ELKSTATE.ELK_ONCOMING_RIGHT;
        IN_R=true;
    end
elseif OverTaking>0 && flag_Onk1==single(0) && flag_rek1==single(0)
        Switch=single(3);
        Line_type=single(1);
        flag_Over=single(1);
    if OverTaking==single(1)
        Left=ELKSTATE.ELK_OVERTAKING_LEFT;
         IN_L=true;
    elseif OverTaking==single(2)
        Right=ELKSTATE.ELK_OVERTAKING_RIGHT;
        IN_R=true;
    end 
elseif Re>0 && flag_Onk1==single(0) && flag_Overk1==single(0)
        Switch=single(1);
        Line_type=single(2);   % re
        flag_re=single(1);
    if Re==single(1)
        Left=ELKSTATE.ELK_ACTIVE_LEFT;
         IN_L=true;
    elseif Re==single(2)
        Right=ELKSTATE.ELK_ACTIVE_RIGHT;
        IN_R=true;
    end 
end

== matlab function PvtSubSys_VSM_ELK/ELK_OnComing_OverTaking/OnComing/MATLAB Function ==
  data: Object_ELKLeftLaneObjType input; LOnComing output; Object_ELKRightLaneObjType input; Object_DX input; Object_DY input; Object_VX input; Object_Width input; Ego_Width input; v input; ROnComing output; Lv_re output; Rv_re output; Lttc output; Rttc output; Llateral output; Rlateral output; la_offset input
function [LOnComing,ROnComing,Lv_re,Rv_re,Lttc,Rttc,Llateral,Rlateral] = fcn(Object_ELKLeftLaneObjType,Object_ELKRightLaneObjType,...
    Object_DX,Object_DY,Object_VX,Object_Width,Ego_Width,v,la_offset)
LOnComing=0;
ROnComing=0;

Lv_re=0;
Rv_re=0;
Lttc=998;
Rttc=998;
Llateral=996;
Rlateral=996;

for  i=1:10
    if Object_ELKLeftLaneObjType(i)==3  % ELKLFOncomingDisMinObj 
            LOnComing=1;
            vx=Object_VX(i);
            dx=Object_DX(i);
            dy=Object_DY(i)-Object_Width(i)-Ego_Width;
            
            Lv_re= abs(vx-v);
            Lttc= dx/ Lv_re;
            Llateral=dy-la_offset;
    end
end
for j=1:10
    if Object_ELKRightLaneObjType(j)==3
            ROnComing=1;
            rvx=Object_VX(j);
            rdx=Object_DX(j);
            rdy=Object_DY(j)+Object_Width(j)+Ego_Width;
            
            Rv_re=abs(rvx-v);
            Rttc=rdx/Rv_re;
            Rlateral=rdy+la_offset;
    end
end

== stateflow chart PvtSubSys_VSM_ELK/ELK_OnComing_OverTaking/OnComing/ONCOMING_FUNCTION ==
  state ONCOMING
    en:on_intervention=0;
  state LEFT_ONCOMING
    en:on_intervention=1;
    LEFT_ONCOMING -> (junction 24) [order 1]
    (junction 24) -> LEFT_ONCOMING [order 1] : [Ldeactive]{left_count = left_count + 1;}
    (junction 24) -> LEFT_ONCOMING [order 2] : {left_count=0;}
  state RIGHT_ONCOMING
    en:on_intervention=2;
    RIGHT_ONCOMING -> (junction 29) [order 1]
    (junction 29) -> RIGHT_ONCOMING [order 1] : [Rdeactive]{right_count = right_count + 1;}
    (junction 29) -> RIGHT_ONCOMING [order 2] : {right_count=0;}
  (default) -> ONCOMING
  ONCOMING -> LEFT_ONCOMING [order 1] : [Leftvalid>0&&Lactive_para&&LOnComing&&Triger]
  LEFT_ONCOMING -> ONCOMING [order 1] : [Leftvalid==0||left_count>50||ELKState<3]{left_count=0;}
  ONCOMING -> RIGHT_ONCOMING [order 2] : [Rightvalid>0&&Ractive_para&&ROnComing&&Triger]
  RIGHT_ONCOMING -> ONCOMING [order 1] : [Rightvalid==0||right_count>50||ELKState<3]{right_count=0;}
  data: LOnComing input; ROnComing input; Leftvalid input; Rightvalid input; Lactive_para input; on_intervention output; Ractive_para input; Ldeactive input; Rdeactive input; left_count local =0; right_count local =0; data local; Triger input; ELKState input

== matlab function PvtSubSys_VSM_ELK/ELK_OnComing_OverTaking/OnComing/OnComing_Judge ==
  data: l_valid input; r_valid input; L_A0 input; L_A1 input; L_A2 input; L_A3 input; R_A0 input; left_condition output; R_A1 input; R_A2 input; R_A3 input; V input; Limit input; Rlimit input; right_condition output; T input; Ldeactive input; Rdeactive input; Out_Offset input; Angle_Offset input; LOut output; ROut output; vehicle_dy input; ifv2bum input; HalfWidth input; LY output; ly output; RY output; ry output; a output
function [left_condition,right_condition,LOut,ROut,LY,ly,RY,ry,a] = fcn(l_valid,r_valid,L_A0,L_A1,L_A2,L_A3,R_A0,R_A1,R_A2,R_A3,V,...
    Limit,Rlimit,T,Ldeactive,Rdeactive,Out_Offset,Angle_Offset,vehicle_dy,ifv2bum,HalfWidth) 
X=V*T;
LY=single(0);
ly=single(0);
RY=single(0);
ry=single(0);
a=single(0);
if l_valid>0
    
   a=atan(L_A1+2*L_A2*X+3*L_A3*X^2);
    if a>0
        ly=(HalfWidth+ifv2bum*tan(a))*cos(a);
    else
        ly=HalfWidth;
    end

   LY=L_A0+L_A1*X+L_A2*X^2+L_A3*X^3;
   left_condition=LY-ly-Limit-vehicle_dy;
   
   if Ldeactive>-Out_Offset && Ldeactive<Out_Offset && abs(atan(L_A1))< Angle_Offset
       LOut=true;  % steady
   else
       LOut=false;
   end       
       
else
    left_condition=single(0);
  LOut=true;
end


if r_valid>0
    
   b=atan(R_A1+2*R_A2*X+3*R_A3*X^2);
    if b<0
        ry=(HalfWidth-ifv2bum*tan(b))*cos(b);
    else
        ry=HalfWidth;
    end

   RY=R_A0+R_A1*X+R_A2*X^2+R_A3*X^3;
   right_condition=RY+ry-Rlimit+vehicle_dy;
   
   if Rdeactive>-Out_Offset && Rdeactive<Out_Offset && abs(atan(R_A1))<Angle_Offset
       ROut=true;
   else
       ROut=false;
   end 
else 
    right_condition=single(0);
    ROut=true;
  
end

== matlab function PvtSubSys_VSM_ELK/ELK_OnComing_OverTaking/OnComing/left_oncoming ==
  data: v input; oncoming output; dx input; inID input; dy input; vx input; lvrel output; lttc output; llateral output; offset input
function [oncoming,lvrel,lttc,llateral] = fcn(v,dx,inID,dy,vx,offset)
t_x=single((-99)*ones(8,1));
t=single(0);
v_t=single(0);
x=single(0);
y=single(99);
for i=1:8
    if inID(i)>0    % left lateral range
        t_x(i)=dx(i);    % related long target
    end
end
for k=1:8
    if t_x(k)>0           % find lateral target
        t=t_x(k);
        break
    end
end
for j=1:8
    if t_x(j) <= t && t_x(j) > -5
        t=t_x(j);      %min(long) target
        v_t=vx(j);
        x=dx(j);
        y=dy(j)-offset(j);
    end
end
if  v_t<0  && abs(v_t) > v  %   in diffrent direction
    oncoming=single(1);
    llateral=y; % dis of taredge to egoedge
    lvrel=-v_t+v-v; 
    lttc=x/lvrel;  
else
    oncoming=single(0);
    llateral=single(988);
    lvrel=single(0);
    lttc=single(999);
end

== matlab function PvtSubSys_VSM_ELK/ELK_OnComing_OverTaking/OnComing/right_oncoming ==
  data: v input; oncoming output; dx input; inID input; dy input; vx input; lvrel output; lttc output; llateral output; offset input
function [oncoming,lvrel,lttc,llateral] = fcn(v,dx,inID,dy,vx,offset)
t_x=single((-99)*ones(8,1));
t=single(0);
v_t=single(0);
x=single(0);
y=single(99);
for i=1:8
    if inID(i)>0     % left lateral range
        t_x(i)=dx(i);    % related long target
    end
end
for k=1:8
    if t_x(k)>0           % find lateral target
        t=t_x(k);
        break
    end
end
for j=1:8
    if t_x(j) <= t && t_x(j) > -5
        t=t_x(j);      %min(long) target
        v_t=vx(j);
        x=dx(j);
        y=dy(j)+offset(j);
    end
end
if  v_t<0  && abs(v_t) > v  %   in diffrent direction
    oncoming=single(1);
    llateral=y;
    lvrel=-v_t+v-v;  
    lttc=x/lvrel;  
else
    oncoming=single(0);
    llateral=single(-988);
    lvrel=single(0);
    lttc=single(999);


end
